simulink library "nlmpclib"  (Simulink 3.00)
values from neighbouring files (symbols this model uses):
  dmodel = modelpd(:,nu+1:nund)    [nlcmpc.m]
  m = ichk(1)    [cmpc.m]    (also in dlqe2.m = dareiter(phi',c',r,gamw*q*gamw'); mod2ss.m = sum(minfo(3:5)); nlcmpc.m = mp(1:max(size(mp))-1); ploteach.m = mu)
  model = ss2mod(a,b,c,d,minfom)    [addmd.m]    (also in nlcmpc.m = modelpd(:,1:nu); tfd2mod.m = ss2mod(a,b,c,d,delt))
  p = sum(no_moves) + nm + 1    [cmpc.m]    (also in dlqe2.m = m-k*c*m; nlcmpc.m = mp(max(size(mp))); paramod.m = sum(minfo1(6:7)); scmpc.m = 1)
  r = zeros(1,ny)    [nlcmpc.m]
  tfilter = tfilter(1,:)    [cmpc.m]
  u0 = zeros(m,1)    [mod2ss.m]    (also in ss2mod.m = u0(:))
  uwt = ryuwt(:,2*ny+1:2*ny+nu)    [nlcmpc.m]    (also in scmpc.m = uwt+10*sqrt(eps))
  ywt = ryuwt(:,ny+1:2*ny)    [nlcmpc.m]    (also in scmpc.m = ones(1,nyi))
undefined symbols (not defined in the file or in its folder): d0, u_lim, y_lim
settings Model: RequirementInfo=9  Creator=greg  LastModifiedBy=eyarrow

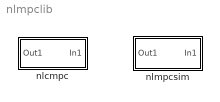
== system nlmpclib ==
  nlcmpc : Subsystem  Orientation=left  mask(CMPC-SIMULINK link){modelpd=[model dmodel], ryuwt=[r ywt uwt], mp=[m p], yulim=[y_lim u_lim], tfilter=tfilter, ud0=[u0 d0]}
      mask help: Masked MATLAB function block calls nlcmpc, links CMPC and SIMULINK.
      mask Help: This links CMPC from MPC-toolbox and SIMULINK. Time must be input into block as last variable in input vector. For information on mask inputs, type help CMPC.
      mask Display: disp('nlcmpc')
  nlmpcsim : Subsystem  Orientation=left  mask(MPCSIM-SIMULINK link){@1=[model dmodel], @2=Kmpc, @3=r, @4=usat, @5=tfilter, @6=[u0 d0]}
      mask prompts: @1 "modelpd:"; @2 "Kmpc:"; @3 "r:"; @4 "usat:"; @5 "tfilter:"; @6 "ud0:"
      mask help: Masked MATLAB function block calls nlmpcsim, links MPCSIM and SIMULINK.
      mask init:
      | modelpd=@1;Kmpc=@2;r=@3;usat=@4;tfilter=@5;ud0=@6;
      mask Help: This links CMPC from MPC-toolbox and SIMULINK. Time must be input into block as last variable in input vector. For information on mask inputs, type help MPCSIM..
      mask Display: disp('nlmpcsim')

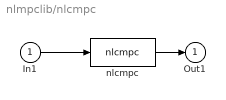
== system nlmpclib/nlcmpc ==
  In1 : Inport  Port=1
  nlcmpc : S-Function  FunctionName=nlcmpc  Parameters=modelpd,mp,tfilter,ryuwt,ud0,yulim  PortCounts=[]  SFunctionModules=''
  Out1 : Outport  Port=1  InitialOutput=0
  wires:
  nlcmpc/1 -> Out1/1
  In1/1 -> nlcmpc/1

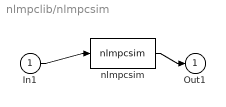
== system nlmpclib/nlmpcsim ==
  In1 : Inport  Port=1
  nlmpcsim : S-Function  FunctionName=nlmpcsim  Parameters=modelpd,Kmpc,r,usat,tfilter,ud0  PortCounts=[]  SFunctionModules=''
  Out1 : Outport  Port=1  InitialOutput=0
  wires:
  nlmpcsim/1 -> Out1/1
  In1/1 -> nlmpcsim/1
